simulink model "sara1_1_restored_from_autosave"  (R2016a)
settings: Solver=ode15s  StartTime=0.0  StopTime=10.0  RelTol=1e-3
values from neighbouring files (symbols this model uses):
  s = a(1)*(t.^3)+a(2)*(t.^2)+a(3)*t+a(4)    [quydao.m]
undefined symbols (not defined in the file or in its folder): gia1, k11, k21, k31, k41, RootGround, RootPart, sara1
libraries: mblibv1 x22, simulink x2
settings Model: Creator=Admin  LastModifiedBy=Admin
settings GRTTargetCC: GeneratePreprocessorConditionals=Use local settings
settings SimMechanicsCC: VisOnUpdateDiagram=on  VisDuringSimulation=on

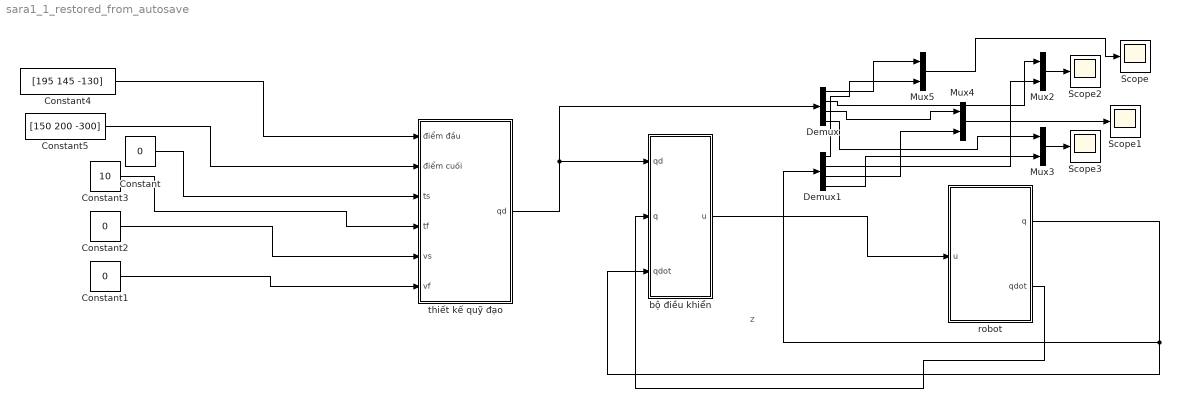
== system sara1_1_restored_from_autosave ==
  note: z
  Constant : Constant  Value=0
  Constant1 : Constant  Value=0
  Constant2 : Constant  Value=0
  Constant3 : Constant  Value=10
  Constant4 : Constant  Value=[195 145 -130]
  Constant5 : Constant  Value=[150 200 -300]
  Demux : Demux
  Demux1 : Demux
  Mux{2..5} (4 alike) : Mux  Inputs=2
  Scope{,1..3} (4 alike) : Scope
  bộ điều khiển : Subsystem
  robot : Subsystem
  thiết kế quỹ đạo : Subsystem
  wires:
  robot/1(q) -> bộ điều khiển/3(qdot), Demux1/1
  Mux2/1 -> Scope2/1
  Mux3/1 -> Scope3/1
  Mux4/1 -> Scope1/1
  Mux5/1 -> Scope/1
  Demux/1 -> Mux5/1
  Demux1/1 -> Mux5/2
  Demux1/2 -> Mux2/2
  Demux/2 -> Mux2/1
  Demux/3 -> Mux4/1
  Demux1/3 -> Mux4/2
  Demux1/4 -> Mux3/2
  Demux/4 -> Mux3/1
  robot/2(qdot) -> bộ điều khiển/2(q)
  bộ điều khiển/1(u) -> robot/1(u)
  thiết kế quỹ đạo/1(qd) -> bộ điều khiển/1(qd), Demux/1
  Constant4/1 -> thiết kế quỹ đạo/1(điểm đầu)
  Constant5/1 -> thiết kế quỹ đạo/2(điểm cuối)
  Constant/1 -> thiết kế quỹ đạo/3(ts)
  Constant3/1 -> thiết kế quỹ đạo/4(tf)
  Constant2/1 -> thiết kế quỹ đạo/5(vs)
  Constant1/1 -> thiết kế quỹ đạo/6(vf)

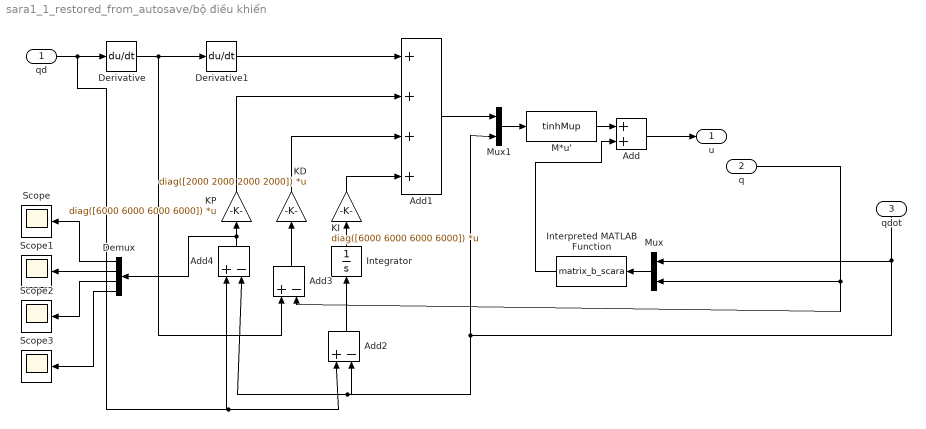
== system sara1_1_restored_from_autosave/bộ điều khiển ==
  qd : Inport
  q : Inport  Port=2
  qdot : Inport  Port=3
  Add : Sum
  Add1 : Sum  Inputs=++++
  Add2 : Sum  Inputs=+|-|
  Add3 : Sum  Inputs=+|-|
  Add4 : Sum  Inputs=+|-|
  Demux : Demux
  Derivative : Derivative
  Derivative1 : Derivative
  Integrator : Integrator
  Interpreted MATLAB Function : MATLABFcn  MATLABFcn=matrix_b_scara  OutputDimensions=4
  KD : Gain  Gain=diag([2000 2000 2000 2000])  Multiplication=Matrix(K*u)
  KI : Gain  Gain=diag([6000 6000 6000 6000])  Multiplication=Matrix(K*u)
  KP : Gain  Gain=diag([6000 6000 6000 6000])  Multiplication=Matrix(K*u)
  M*u' : MATLABFcn  MATLABFcn=tinhMup  OutputDimensions=4
  Mux : Mux  Inputs=2
  Mux1 : Mux  Inputs=2
  Scope{,1..3} (4 alike) : Scope
  u : Outport
  wires:
  qdot/1 -> Add4/2, Add2/2, Mux1/2, Mux/1
  qd/1 -> Add4/1, Add2/1, Derivative/1
  Interpreted MATLAB Function/1 -> Add/2
  Mux/1 -> Interpreted MATLAB Function/1
  Derivative1/1 -> Add1/1
  Add/1 -> u/1
  KP/1 -> Add1/2
  Integrator/1 -> KI/1
  Add2/1 -> Integrator/1
  Add3/1 -> KD/1
  Add4/1 -> Demux/1, KP/1
  KD/1 -> Add1/3
  Derivative/1 -> Add3/1, Derivative1/1
  q/1 -> Add3/2, Mux/2
  M*u'/1 -> Add/1
  Add1/1 -> Mux1/1
  Mux1/1 -> M*u'/1
  KI/1 -> Add1/4
  Demux/1 -> Scope/1
  Demux/2 -> Scope1/1
  Demux/3 -> Scope2/1
  Demux/4 -> Scope3/1

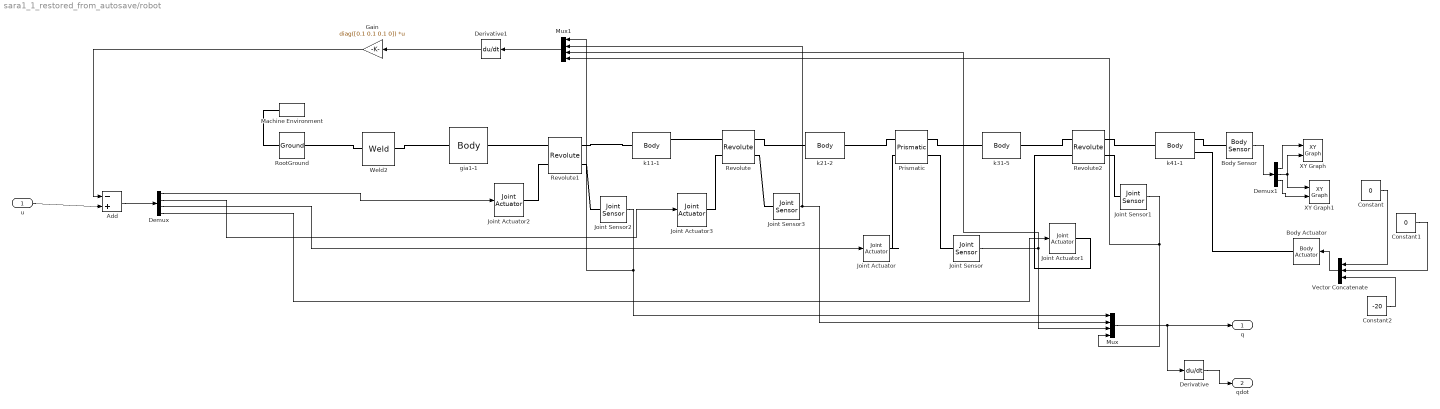
== system sara1_1_restored_from_autosave/robot ==
  u : Inport
  Add : Sum  Inputs=-|+|
  Body Actuator : mblibv1/Sensors &  Actuators/Body Actuator  UpdateFromCAD=off  PhysicalDomain=Mechanical  PortType=blob  ActuationStyle=Force  AngleUnits=deg  ArcVelocityUnits=deg/s  ArcAccelerationUnits=deg/s^2  CoordPositionUnits=m  VelocityUnits=m/s  AccelerationUnits=m/s^2  ForceUnits=N  TorqueUnits=N-m  ActiveIO=on  Width=3  DialogClass=MechanicalActuatorBlock  ReferenceFrame=Absolute (World)  Angle=off  CoordPosition=on  Force=on  Torque=off
  Body Sensor : mblibv1/Sensors &  Actuators/Body Sensor  UpdateFromCAD=off  PhysicalDomain=Mechanical  PortType=blob  Muxed=on  Pose=off  Angle=on  AngleUnits=deg  ArcVelocity=off  ArcVelocityUnits=deg/s  ArcAcceleration=off  ArcAccelerationUnits=deg/s^2  CoordPosition=on  CoordPositionUnits=mm  Velocity=off  VelocityUnits=m/s  Acceleration=off  AccelerationUnits=m/s^2  Quaternion=on  QuaternionDT=off  QuaternionDDT=off  QuaternionUnits=off  OutputVector=[1]  ActiveIO=on  Width=3  DialogClass=MechanicalSensorBlock  ReferenceFrame=Absolute (World)
  Constant : Constant  Value=0
  Constant1 : Constant  Value=0
  Constant2 : Constant  Value=-20
  Demux : Demux
  Demux1 : Demux  Outputs=3
  Derivative : Derivative
  Derivative1 : Derivative
  Gain : Gain  Gain=diag([0.1 0.1 0.1 0])  Multiplication=Matrix(K*u)
  Joint Actuator : mblibv1/Sensors &  Actuators/Joint Actuator  UpdateFromCAD=off  PhysicalDomain=Mechanical  PortType=blob  ActuationStyle=Force  AngleUnits=deg  ArcVelocityUnits=deg/s  ArcAccelerationUnits=deg/s^2  CoordPositionUnits=m  VelocityUnits=m/s  AccelerationUnits=m/s^2  ForceUnits=N  TorqueUnits=N-m  ActiveIO=on  Width=1  DialogClass=MechanicalActuatorBlock  Primitive=P1  ReferenceFrame=Absolute (World)
  Joint Actuator1 : mblibv1/Sensors &  Actuators/Joint Actuator  UpdateFromCAD=off  PhysicalDomain=Mechanical  PortType=blob  ActuationStyle=Force  AngleUnits=deg  ArcVelocityUnits=deg/s  ArcAccelerationUnits=deg/s^2  CoordPositionUnits=m  VelocityUnits=m/s  AccelerationUnits=m/s^2  ForceUnits=N  TorqueUnits=N-m  ActiveIO=on  Width=1  DialogClass=MechanicalActuatorBlock  Primitive=R1  ReferenceFrame=Absolute (World)
  Joint Actuator2 : mblibv1/Sensors &  Actuators/Joint Actuator  UpdateFromCAD=off  PhysicalDomain=Mechanical  PortType=blob  ActuationStyle=Force  AngleUnits=deg  ArcVelocityUnits=deg/s  ArcAccelerationUnits=deg/s^2  CoordPositionUnits=m  VelocityUnits=m/s  AccelerationUnits=m/s^2  ForceUnits=N  TorqueUnits=N-m  ActiveIO=on  Width=1  DialogClass=MechanicalActuatorBlock  Primitive=R1  ReferenceFrame=Absolute (World)
  Joint Actuator3 : mblibv1/Sensors &  Actuators/Joint Actuator  UpdateFromCAD=off  PhysicalDomain=Mechanical  PortType=blob  ActuationStyle=Force  AngleUnits=deg  ArcVelocityUnits=deg/s  ArcAccelerationUnits=deg/s^2  CoordPositionUnits=m  VelocityUnits=m/s  AccelerationUnits=m/s^2  ForceUnits=N  TorqueUnits=N-m  ActiveIO=on  Width=1  DialogClass=MechanicalActuatorBlock  Primitive=R1  ReferenceFrame=Absolute (World)
  Joint Sensor : mblibv1/Sensors &  Actuators/Joint Sensor  UpdateFromCAD=off  PhysicalDomain=Mechanical  PortType=blob  Muxed=on  Pose=off  Angle=on  AngleUnits=deg  ArcVelocity=off  ArcVelocityUnits=deg/s  ArcAcceleration=off  ArcAccelerationUnits=deg/s^2  CoordPosition=on  CoordPositionUnits=m  Velocity=off  VelocityUnits=m/s  Acceleration=off  AccelerationUnits=m/s^2  Quaternion=on  QuaternionDT=off  QuaternionDDT=off  QuaternionUnits=off  OutputVector=[1]  ActiveIO=on  Width=1  DialogClass=MechanicalSensorBlock  Primitive=P1  Force=off  ForceUnits=N  Torque=off  TorqueUnits=N-m  ReferenceFrame=Absolute (World)  ReactionSensedSide=Base  ReactionReferenceFrame=Absolute (World)  ReactionForce=off  ReactionForceUnits=N  ReactionMoment=off  ReactionMomentUnits=N-m
  Joint Sensor1 : mblibv1/Sensors &  Actuators/Joint Sensor  UpdateFromCAD=off  PhysicalDomain=Mechanical  PortType=blob  Muxed=on  Pose=off  Angle=on  AngleUnits=rad  ArcVelocity=off  ArcVelocityUnits=deg/s  ArcAcceleration=off  ArcAccelerationUnits=deg/s^2  CoordPosition=on  CoordPositionUnits=m  Velocity=off  VelocityUnits=m/s  Acceleration=off  AccelerationUnits=m/s^2  Quaternion=on  QuaternionDT=off  QuaternionDDT=off  QuaternionUnits=off  OutputVector=[1]  ActiveIO=on  Width=1  DialogClass=MechanicalSensorBlock  Primitive=R1  Force=off  ForceUnits=N  Torque=off  TorqueUnits=N*m  ReferenceFrame=Absolute (World)  ReactionSensedSide=Base  ReactionReferenceFrame=Absolute (World)  ReactionForce=off  ReactionForceUnits=N  ReactionMoment=off  ReactionMomentUnits=N*m
  Joint Sensor2 : mblibv1/Sensors &  Actuators/Joint Sensor  UpdateFromCAD=off  PhysicalDomain=Mechanical  PortType=blob  Muxed=on  Pose=off  Angle=on  AngleUnits=rad  ArcVelocity=off  ArcVelocityUnits=rad/s  ArcAcceleration=off  ArcAccelerationUnits=deg/s^2  CoordPosition=on  CoordPositionUnits=m  Velocity=off  VelocityUnits=m/s  Acceleration=off  AccelerationUnits=m/s^2  Quaternion=on  QuaternionDT=off  QuaternionDDT=off  QuaternionUnits=off  OutputVector=[1]  ActiveIO=on  Width=1  DialogClass=MechanicalSensorBlock  Primitive=R1  Force=off  ForceUnits=N  Torque=off  TorqueUnits=N*m  ReferenceFrame=Absolute (World)  ReactionSensedSide=Base  ReactionReferenceFrame=Absolute (World)  ReactionForce=off  ReactionForceUnits=N  ReactionMoment=off  ReactionMomentUnits=N*m
  Joint Sensor3 : mblibv1/Sensors &  Actuators/Joint Sensor  UpdateFromCAD=off  PhysicalDomain=Mechanical  PortType=blob  Muxed=on  Pose=off  Angle=on  AngleUnits=rad  ArcVelocity=off  ArcVelocityUnits=deg/s  ArcAcceleration=off  ArcAccelerationUnits=deg/s^2  CoordPosition=on  CoordPositionUnits=m  Velocity=off  VelocityUnits=m/s  Acceleration=off  AccelerationUnits=m/s^2  Quaternion=on  QuaternionDT=off  QuaternionDDT=off  QuaternionUnits=off  OutputVector=[1]  ActiveIO=on  Width=1  DialogClass=MechanicalSensorBlock  Primitive=R1  Force=off  ForceUnits=N  Torque=off  TorqueUnits=N*m  ReferenceFrame=Absolute (World)  ReactionSensedSide=Base  ReactionReferenceFrame=Absolute (World)  ReactionForce=off  ReactionForceUnits=N  ReactionMoment=off  ReactionMomentUnits=N*m
  Machine Environment : mblibv1/Bodies/Machine Environment  PortType=env  PhysicalDomain=Mechanical  DialogTemplateClass=MECH.MachineEnvironment  SyncWhenCopied=off  Gravity=[0 0 -9.81]  GravityUnits=m/s^2  GravityAsSignal=off  Dimensionality=Auto-detect  AnalysisType=Forward dynamics  LinearAssemblyTolerance=1e-3  LinearAssemblyToleranceUnits=m  AngularAssemblyTolerance=1e-3  AngularAssemblyToleranceUnits=rad  ConstraintSolverType=Stabilizing  ConstraintRelTolerance=1e-4  ConstraintAbsTolerance=1e-4  UseRobustSingularityHandling=off  RedundancyAnalysisToleranceType=Automatically select tolerance  RedundancyAnalysisTolerance=1e-14  StatePerturbationType=Fixed  PerturbationSize=1e-5  VisualizeMachine=on  BodyVisualizationType=Use model default body geometries  BodyColorSelMode=Use model default  DefaultBodyColor=[1 0 0]
  Mux : Mux
  Mux1 : Mux
  Prismatic : mblibv1/Joints/Prismatic  LConnTagsString=__newl0|SA1  RConnTagsString=__newr0|SA1  UpdateFromCAD=on  PMImportedID=k21-2:-:k31-5  NumSAPorts=2  CutJoint=off  MarkAsCut=off  Primitives=prismatic  PrimitiveProps=P1$Base$[0,0,1]$prismatic  DialogClass=JointBlock  P1Axis=[0,0,1]
  Revolute : mblibv1/Joints/Revolute  LConnTagsString=__newl0|SA1  RConnTagsString=__newr0|SA1  UpdateFromCAD=on  PMImportedID=k11-1:-:k21-2  NumSAPorts=2  CutJoint=off  MarkAsCut=off  Primitives=prismatic  PrimitiveProps=R1$Base$[0,0,1]$revolute  DialogClass=JointBlock  R1Axis=[0,0,1]
  Revolute1 : mblibv1/Joints/Revolute  LConnTagsString=__newl0|SA1  RConnTagsString=__newr0|SA1  UpdateFromCAD=on  PMImportedID=gia1-1:-:k11-1  NumSAPorts=2  CutJoint=off  MarkAsCut=off  Primitives=prismatic  PrimitiveProps=R1$Base$[0,0,1]$revolute  DialogClass=JointBlock  R1Axis=[0,0,1]
  Revolute2 : mblibv1/Joints/Revolute  LConnTagsString=__newl0|SA1  RConnTagsString=__newr0|SA1  UpdateFromCAD=on  PMImportedID=k31-5:-:k41-1  NumSAPorts=2  CutJoint=off  MarkAsCut=off  Primitives=prismatic  PrimitiveProps=R1$Base$[0,0,1]$revolute  DialogClass=JointBlock  R1Axis=[0,0,1]
  RootGround : mblibv1/Bodies/Ground  UpdateFromCAD=on  PMImportedID=RootGround  LeftPortType=env  RightPortType=workingframe  PhysicalDomain=Mechanical  DialogClass=GroundBlock  CoordPosition=[0 0 0]  CoordPositionUnits=m  StateVectorMgrId=2  MachineId=[3 0]  ShowEnvPort=on  ParameterChecksum=[3431329664, 1919006669, 890914081, 1826314844]  TopologyChecksum=[1642285356, 382317968, 2627216132, 3125865323]
  Vector Concatenate : Concatenate  NumInputs=3
  Weld2 : mblibv1/Joints/Weld  LConnTagsString=__newl0  RConnTagsString=__newr0  UpdateFromCAD=on  PMImportedID=RootGround:-:sara1/RootPart  NumSAPorts=0  CutJoint=off  MarkAsCut=off  Primitives=weld  PrimitiveProps=W$World$[0.57735,0.57735,0.57735]$weld  DialogClass=JointBlock  WAxis=[0.57735,0.57735,0.57735]
  XY Graph : simulink/Sinks/XY Graph  xmin=100  xmax=250  ymin=100  ymax=250  st=-1
  XY Graph1 : simulink/Sinks/XY Graph  xmin=100  xmax=250  ymin=-350  ymax=-100  st=-1
  gia1-1 : mblibv1/Bodies/Body  LConnTagsString=CS2  RConnTagsString=CS4  UpdateFromCAD=on  PMImportedID=gia1-1  DialogClass=MechanicalBodyBlock  Mass=7  MassUnits=kg  InertiaUnits=kg*m^2  Inertia=[0.0144639,0,0;0,0.0144639,0;0,0,0.000297178]  Shape=Cylinder  ShapeDims=[1 1]  ShapeUnits=m  ShapeUse=false  Density=1  DensityUnits=kg/m^3  DensityUse=false  GraphicsMode=GFXFILE  GraphicsFileName=sara1 - gia1-1.STL  BodyColorSelMode=COLORPALETTE  BodyColor=[0.098039 0.79216 1]  AttachedToCS=CS1  CG=Right$CG$[0 0 -0.277667]$WORLD$WORLD$m$[1 0 0;0 1 0;0 0 1]$3x3 Transform$rad$WORLD$false$gia1-1::CG(AUTOGEN)  WorkingFrames=Right$CS1$[0 0 -0.4]$WORLD$WORLD$m$[1 0 0;0 1 0;0 0 1]$3x3 Transform$rad$WORLD$false$gia1-1::CS1(AUTOGEN)#Left$CS2$[0 0 0]$WORLD$WORLD$m$[1 0 0;0 1 0;0 0 1]$3x3 Transform$rad$WORLD$true$gia1-1:-:sara1/RootPart::gia1-1(AUTOGEN)#Right$CS4$[0 0 0]$WORLD$WORLD$m$[1 0 0;0 1 0;0 0 1]$3x3 Transform$rad$WORLD$true$gia1-1:-:k11-1::gia1-1(AUTOGEN)  CGPos=[0 0 -0.277667]  CGRot=[1 0 0;0 1 0;0 0 1]  CS0Pos=[]  CS0Rot=[]  CS1Pos=[0 0 -0.4]  CS1Rot=[1 0 0;0 1 0;0 0 1]  CS2Pos=[0 0 0]  CS2Rot=[1 0 0;0 1 0;0 0 1]  CS3Pos=[]  CS3Rot=[]  CS4Pos=[0 0 0]  CS4Rot=[1 0 0;0 1 0;0 0 1]  CS5Pos=[]  CS5Rot=[]  CS6Pos=[]  CS6Rot=[]  CS7Pos=[]  CS7Rot=[]  CS8Pos=[]  CS8Rot=[]  CS9Pos=[]  CS9Rot=[]  CS10Pos=[]  CS10Rot=[]  CS11Pos=[]  CS11Rot=[]  CS12Pos=[]  CS12Rot=[]  CS13Pos=[]  CS13Rot=[]  CS14Pos=[]  CS14Rot=[]  CS15Pos=[]  CS15Rot=[]  CS16Pos=[]  CS16Rot=[]  CS17Pos=[]  CS17Rot=[]  CS18Pos=[]  CS18Rot=[]  CS19Pos=[]  CS19Rot=[]  CS20Pos=[]  CS20Rot=[]
  k11-1 : mblibv1/Bodies/Body  LConnTagsString=CS3  RConnTagsString=CS2|CS4  UpdateFromCAD=on  PMImportedID=k11-1  DialogClass=MechanicalBodyBlock  Mass=6  MassUnits=kg  InertiaUnits=kg*m^2  Inertia=[0.0001 0 0; 0 0.0190125 0; 0 0 0.0190125]  Shape=Cylinder  ShapeDims=[1 1]  ShapeUnits=m  ShapeUse=false  Density=1  DensityUnits=kg/m^3  DensityUse=false  GraphicsMode=GFXFILE  GraphicsFileName=sara1 - k11-1.STL  BodyColorSelMode=COLORPALETTE  BodyColor=[1 0 0]  AttachedToCS=CS1  CG=Right$CG$[0.0975 0 0]$CS3$CS3$m$[1 0 0;0 1 0;0 0 1]$3x3 Transform$rad$WORLD$false$k11-1::CG(AUTOGEN)  WorkingFrames=Right$CS1$[0.0975 0 -0.02]$WORLD$WORLD$m$[1 0 0;0 1 0;0 0 1]$3x3 Transform$rad$WORLD$false$k11-1::CS1(AUTOGEN)#Right$CS2$[0.195 0 0]$WORLD$WORLD$m$[1 0 0;0 1 0;0 0 1]$3x3 Transform$rad$WORLD$true$k11-1:-:k21-2::k11-1(AUTOGEN)#Right$CS4$[0.195 0 0]$WORLD$WORLD$m$[1 0 0;0 1 0;0 0 1]$3x3 Transform$rad$WORLD$true$none#Left$CS3$[0 0 0]$WORLD$WORLD$m$[1 0 0;0 1 0;0 0 1]$3x3 Transform$rad$WORLD$true$gia1-1:-:k11-1::k11-1(AUTOGEN)  CGPos=[0.0975 0 0]  CGRot=[1 0 0;0 1 0;0 0 1]  CS0Pos=[]  CS0Rot=[]  CS1Pos=[0.0975 0 -0.02]  CS1Rot=[1 0 0;0 1 0;0 0 1]  CS2Pos=[0.195 0 0]  CS2Rot=[1 0 0;0 1 0;0 0 1]  CS3Pos=[0 0 0]  CS3Rot=[1 0 0;0 1 0;0 0 1]  CS4Pos=[0.195 0 0]  CS4Rot=[1 0 0;0 1 0;0 0 1]  CS5Pos=[]  CS5Rot=[]  CS6Pos=[]  CS6Rot=[]  CS7Pos=[]  CS7Rot=[]  CS8Pos=[]  CS8Rot=[]  CS9Pos=[]  CS9Rot=[]  CS10Pos=[]  CS10Rot=[]  CS11Pos=[]  CS11Rot=[]  CS12Pos=[]  CS12Rot=[]  CS13Pos=[]  CS13Rot=[]  CS14Pos=[]  CS14Rot=[]  CS15Pos=[]  CS15Rot=[]  CS16Pos=[]  CS16Rot=[]  CS17Pos=[]  CS17Rot=[]  CS18Pos=[]  CS18Rot=[]  CS19Pos=[]  CS19Rot=[]  CS20Pos=[]  CS20Rot=[]
  k21-2 : mblibv1/Bodies/Body  LConnTagsString=CS2  RConnTagsString=CS3  UpdateFromCAD=on  PMImportedID=k21-2  DialogClass=MechanicalBodyBlock  Mass=5  MassUnits=kg  InertiaUnits=kg*m^2  Inertia=[0.00012 0 0; 0 0.008760416667 0; 0 0 0.008760416667]  Shape=Cylinder  ShapeDims=[1 1]  ShapeUnits=m  ShapeUse=false  Density=1  DensityUnits=kg/m^3  DensityUse=false  GraphicsMode=GFXFILE  GraphicsFileName=sara1 - k21-2.STL  BodyColorSelMode=COLORPALETTE  BodyColor=[1 1 0]  AttachedToCS=CS1  CG=Right$CG$[0 0.0725 0]$CS2$CS2$m$[0 1 0;1 0 0;0 0 -1]$3x3 Transform$rad$WORLD$false$k21-2::CG(AUTOGEN)  WorkingFrames=Right$CS1$[0.195 0.0725 0]$WORLD$WORLD$m$[0 -1 0;1 0 0;0 0 1]$3x3 Transform$rad$WORLD$false$k21-2::CS1(AUTOGEN)#Left$CS2$[0.195 0 0]$WORLD$WORLD$m$[1 0 0;0 1 0;0 0 1]$3x3 Transform$rad$WORLD$true$k11-1:-:k21-2::k21-2(AUTOGEN)#Right$CS3$[0.195 0.145 0]$WORLD$WORLD$m$[0 1 0;1 0 0;0 0 -1]$3x3 Transform$rad$WORLD$true$k21-2:-:k31-5::k21-2(AUTOGEN)  CGPos=[0 0.0725 0]  CGRot=[0 1 0;1 0 0;0 0 -1]  CS0Pos=[]  CS0Rot=[]  CS1Pos=[0.195 0.0725 0]  CS1Rot=[0 -1 0;1 0 0;0 0 1]  CS2Pos=[0.195 0 0]  CS2Rot=[1 0 0;0 1 0;0 0 1]  CS3Pos=[0.195 0.145 0]  CS3Rot=[0 1 0;1 0 0;0 0 -1]  CS4Pos=[]  CS4Rot=[]  CS5Pos=[]  CS5Rot=[]  CS6Pos=[]  CS6Rot=[]  CS7Pos=[]  CS7Rot=[]  CS8Pos=[]  CS8Rot=[]  CS9Pos=[]  CS9Rot=[]  CS10Pos=[]  CS10Rot=[]  CS11Pos=[]  CS11Rot=[]  CS12Pos=[]  CS12Rot=[]  CS13Pos=[]  CS13Rot=[]  CS14Pos=[]  CS14Rot=[]  CS15Pos=[]  CS15Rot=[]  CS16Pos=[]  CS16Rot=[]  CS17Pos=[]  CS17Rot=[]  CS18Pos=[]  CS18Rot=[]  CS19Pos=[]  CS19Rot=[]  CS20Pos=[]  CS20Rot=[]
  k31-5 : mblibv1/Bodies/Body  LConnTagsString=CS2  RConnTagsString=CS3  UpdateFromCAD=on  PMImportedID=k31-5  DialogClass=MechanicalBodyBlock  Mass=4  MassUnits=kg  InertiaUnits=kg*m^2  Inertia=[0.02083333333 0 0; 0 0.02083333333 0; 0 0 0.00014;]  Shape=Cylinder  ShapeDims=[1 1]  ShapeUnits=m  ShapeUse=false  Density=1  DensityUnits=kg/m^3  DensityUse=false  GraphicsMode=GFXFILE  GraphicsFileName=sara1 - k31-5.STL  BodyColorSelMode=COLORPALETTE  BodyColor=[0 1 0]  AttachedToCS=CS1  CG=Right$CG$[0 0 -0.125]$CS2$CS2$m$[0 1 0;1 0 0;0 0 -1]$3x3 Transform$rad$WORLD$false$k31-5::CG(AUTOGEN)  WorkingFrames=Right$CS1$[0.195 0.145 0.29]$WORLD$WORLD$m$[0 0 1;1 0 0;0 1 0]$3x3 Transform$rad$WORLD$false$k31-5::CS1(AUTOGEN)#Left$CS2$[0.195 0.145 0]$WORLD$WORLD$m$[0 1 0;1 0 0;0 0 -1]$3x3 Transform$rad$WORLD$true$k21-2:-:k31-5::k31-5(AUTOGEN)#Right$CS3$[0.195 0.145 0]$WORLD$WORLD$m$[0 1 0;1 0 0;0 0 -1]$3x3 Transform$rad$WORLD$true$k31-5:-:k41-1::k31-5(AUTOGEN)  CGPos=[0 0 -0.125]  CGRot=[0 1 0;1 0 0;0 0 -1]  CS0Pos=[]  CS0Rot=[]  CS1Pos=[0.195 0.145 0.29]  CS1Rot=[0 0 1;1 0 0;0 1 0]  CS2Pos=[0.195 0.145 0]  CS2Rot=[0 1 0;1 0 0;0 0 -1]  CS3Pos=[0.195 0.145 0]  CS3Rot=[0 1 0;1 0 0;0 0 -1]  CS4Pos=[]  CS4Rot=[]  CS5Pos=[]  CS5Rot=[]  CS6Pos=[]  CS6Rot=[]  CS7Pos=[]  CS7Rot=[]  CS8Pos=[]  CS8Rot=[]  CS9Pos=[]  CS9Rot=[]  CS10Pos=[]  CS10Rot=[]  CS11Pos=[]  CS11Rot=[]  CS12Pos=[]  CS12Rot=[]  CS13Pos=[]  CS13Rot=[]  CS14Pos=[]  CS14Rot=[]  CS15Pos=[]  CS15Rot=[]  CS16Pos=[]  CS16Rot=[]  CS17Pos=[]  CS17Rot=[]  CS18Pos=[]  CS18Rot=[]  CS19Pos=[]  CS19Rot=[]  CS20Pos=[]  CS20Rot=[]
  k41-1 : mblibv1/Bodies/Body  LConnTagsString=CS2  RConnTagsString=CS3|CS4  UpdateFromCAD=on  PMImportedID=k41-1  DialogClass=MechanicalBodyBlock  Mass=2  MassUnits=kg  InertiaUnits=kg*m^2  Inertia=[0.002816666667 0 0; 0 0.002816666667 0; 0 0 0.00001]  Shape=Cylinder  ShapeDims=[1 1]  ShapeUnits=m  ShapeUse=false  Density=1  DensityUnits=kg/m^3  DensityUse=false  GraphicsMode=GFXFILE  GraphicsFileName=sara1 - k41-1.STL  BodyColorSelMode=COLORPALETTE  BodyColor=[0.79216 0.81961 0.93333]  AttachedToCS=CS1  CG=Right$CG$[0 0 0.065]$CS2$CS2$m$[0 1 0;1 0 0;0 0 -1]$3x3 Transform$rad$WORLD$false$k41-1::CG(AUTOGEN)  WorkingFrames=Right$CS1$[0.195 0.145 -0.12]$WORLD$WORLD$m$[0 -1 0;1 0 0;0 0 1]$3x3 Transform$rad$WORLD$false$k41-1::CS1(AUTOGEN)#Right$CS3$[0.195 0.145 -0.13]$WORLD$WORLD$m$[0 1 0;1 0 0;0 0 -1]$3x3 Transform$rad$WORLD$true$none#Right$CS4$[0.195 0.145 -0.13]$WORLD$WORLD$m$[0 1 0;1 0 0;0 0 -1]$3x3 Transform$rad$WORLD$true$none#Left$CS2$[0.195 0.145 0]$WORLD$WORLD$m$[0 1 0;1 0 0;0 0 -1]$3x3 Transform$rad$WORLD$true$k31-5:-:k41-1::k41-1(AUTOGEN)  CGPos=[0 0 0.065]  CGRot=[0 1 0;1 0 0;0 0 -1]  CS0Pos=[]  CS0Rot=[]  CS1Pos=[0.195 0.145 -0.12]  CS1Rot=[0 -1 0;1 0 0;0 0 1]  CS2Pos=[0.195 0.145 0]  CS2Rot=[0 1 0;1 0 0;0 0 -1]  CS3Pos=[0.195 0.145 -0.13]  CS3Rot=[0 1 0;1 0 0;0 0 -1]  CS4Pos=[0.195 0.145 -0.13]  CS4Rot=[0 1 0;1 0 0;0 0 -1]  CS5Pos=[]  CS5Rot=[]  CS6Pos=[]  CS6Rot=[]  CS7Pos=[]  CS7Rot=[]  CS8Pos=[]  CS8Rot=[]  CS9Pos=[]  CS9Rot=[]  CS10Pos=[]  CS10Rot=[]  CS11Pos=[]  CS11Rot=[]  CS12Pos=[]  CS12Rot=[]  CS13Pos=[]  CS13Rot=[]  CS14Pos=[]  CS14Rot=[]  CS15Pos=[]  CS15Rot=[]  CS16Pos=[]  CS16Rot=[]  CS17Pos=[]  CS17Rot=[]  CS18Pos=[]  CS18Rot=[]  CS19Pos=[]  CS19Rot=[]  CS20Pos=[]  CS20Rot=[]
  q : Outport
  qdot : Outport  Port=2
  wires:
  Joint Sensor3/1 -> Mux/2, Mux1/2
  Joint Sensor1/1 -> Mux1/4, Mux/4
  Demux/1 -> Joint Actuator2/1
  Demux/2 -> Joint Actuator3/1
  Demux/3 -> Joint Actuator/1
  Demux/4 -> Joint Actuator1/1
  Joint Sensor2/1 -> Mux1/1, Mux/1
  Joint Sensor/1 -> Mux1/3, Mux/3
  Mux/1 -> Derivative/1, q/1
  Derivative/1 -> qdot/1
  u/1 -> Add/2
  Body Sensor/1 -> Demux1/1
  Demux1/1 -> XY Graph/1
  Demux1/2 -> XY Graph/2, XY Graph1/1
  Demux1/3 -> XY Graph1/2
  Vector Concatenate/1 -> Body Actuator/1
  Constant2/1 -> Vector Concatenate/3
  Constant1/1 -> Vector Concatenate/2
  Constant/1 -> Vector Concatenate/1
  Mux1/1 -> Derivative1/1
  Derivative1/1 -> Gain/1
  Gain/1 -> Add/1
  Add/1 -> Demux/1
  connections:
  Revolute2/RConn1 -- k41-1/LConn1
  Prismatic/RConn2 -- Joint Sensor/LConn1
  Joint Actuator1/RConn1 -- Revolute2/LConn2
  Joint Sensor3/LConn1 -- Revolute/RConn2
  Joint Actuator3/RConn1 -- Revolute/LConn2
  Revolute/RConn1 -- k21-2/LConn1
  k21-2/RConn1 -- Prismatic/LConn1
  Prismatic/RConn1 -- k31-5/LConn1
  Revolute1/RConn1 -- k11-1/LConn1
  RootGround/RConn1 -- Weld2/LConn1
  gia1-1/RConn1 -- Revolute1/LConn1
  gia1-1/LConn1 -- Weld2/RConn1
  k11-1/RConn1 -- Revolute/LConn1
  RootGround/LConn1 -- Machine Environment/RConn1
  Joint Actuator/RConn1 -- Prismatic/LConn2
  Revolute2/RConn2 -- Joint Sensor1/LConn1
  k31-5/RConn1 -- Revolute2/LConn1
  Body Sensor/LConn1 -- k41-1/RConn1
  Body Actuator/RConn1 -- k41-1/RConn2
  Joint Actuator2/RConn1 -- Revolute1/LConn2
  Joint Sensor2/LConn1 -- Revolute1/RConn2

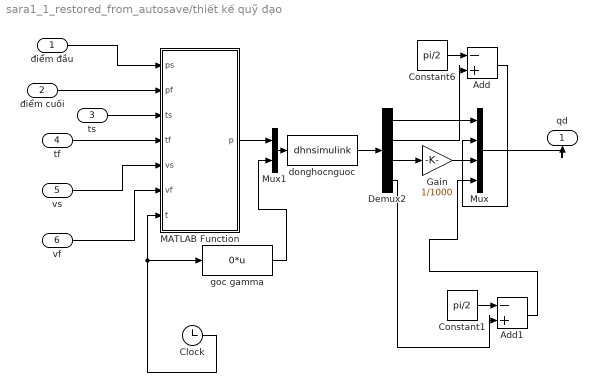
== system sara1_1_restored_from_autosave/thiết kế quỹ đạo ==
  điểm đầu : Inport
  điểm cuối : Inport  Port=2
  ts : Inport  Port=3
  tf : Inport  Port=4
  vs : Inport  Port=5
  vf : Inport  Port=6
  Add : Sum  Inputs=-|+|
  Add1 : Sum  Inputs=-|+|
  Clock : Clock
  Constant1 : Constant  Value=pi/2
  Constant6 : Constant  Value=pi/2
  Demux2 : Demux
  Gain : Gain  Gain=1/1000
  MATLAB Function : MATLAB Function  TreatAsAtomicUnit=on
  Mux : Mux
  Mux1 : Mux  Inputs=2
  donghocnguoc : MATLABFcn  MATLABFcn=dhnsimulink  OutputDimensions=4
  goc gamma : MATLABFcn  MATLABFcn=0*u
  qd : Outport
  wires:
  Clock/1 -> MATLAB Function/7(t), goc gamma/1
  Mux1/1 -> donghocnguoc/1
  Constant6/1 -> Add/1
  ts/1 -> MATLAB Function/3(ts)
  vs/1 -> MATLAB Function/5(vs)
  goc gamma/1 -> Mux1/2
  điểm đầu/1 -> MATLAB Function/1(ps)
  tf/1 -> MATLAB Function/4(tf)
  điểm cuối/1 -> MATLAB Function/2(pf)
  Add/1 -> Mux/2
  vf/1 -> MATLAB Function/6(vf)
  MATLAB Function/1(p) -> Mux1/1
  Mux/1 -> qd/1
  Gain/1 -> Mux/3
  Demux2/3 -> Gain/1
  donghocnguoc/1 -> Demux2/1
  Demux2/1 -> Mux/1
  Demux2/2 -> Add/2
  Constant1/1 -> Add1/1
  Add1/1 -> Mux/4
  Demux2/4 -> Add1/2

== matlab function sara1_1_restored_from_autosave/thiết kế quỹ đạo/MATLAB Function ==
  data: ps input; p output; pf input; ts input; tf input; vs input; vf input; t input
% thiet ke quy dao robot duong thang da thuc bac 3
function p=quydaothang(ps,pf,ts,tf,vs,vf,t)
A=[ts^3 ts^2 ts 1;3*ts^2 2*ts 1 0; tf^3 tf^2 tf 1;3*tf^2 2*tf 1 0];
b=[0;vs;sqrt((pf(1)-ps(1))^2+(pf(2)-ps(2))^2+(pf(3)-ps(3))^2);vf];
a=inv(A)*b;
s=a(1)*(t.^3)+a(2)*(t.^2)+a(3)*t+a(4);
p1=ps(1)+(s/sqrt((pf(1)-ps(1))^2+(pf(2)-ps(2))^2+(pf(3)-ps(3))^2))*(pf(1)-ps(1));
p2=ps(2)+(s/sqrt((pf(1)-ps(1))^2+(pf(2)-ps(2))^2+(pf(3)-ps(3))^2))*(pf(2)-ps(2));
p3=ps(3)+(s/sqrt((pf(1)-ps(1))^2+(pf(2)-ps(2))^2+(pf(3)-ps(3))^2))*(pf(3)-ps(3));
p=[p1;p2;p3];
